simulink model "mrefrobotarm_modified_previous_y_previous_u_previous_ref_prepro"  (R2018b)
settings: Solver=FixedStepAuto  StartTime=0.0  StopTime=10  RelTol=1e-3  AbsTol=1e-6
undefined symbols (not defined in the file or in its folder): cc, options
libraries: neural x594, simulink x1
(part 18 of 22)

== system mrefrobotarm_modified_previous_y_previous_u_previous_ref_prepro/pre_0.0001/Layer 3/Delays 1 ==
  "p{3}" : Inport  PortDimensions=30
      mask Display: e = 0.06;c1 = [120 230 180]/255;c2 = ([120 230 180]+0)/(256+128);c3 = ([120 230 180]+128)/(256+128);patch([0 1 1 0],[0 0 1 1],c1);patch([0 1 1 1-e 1-e 0+e],[0 0 1 1-e 0+e 0+e],c2);patch([0 0 1 1-e 0+e 0+e],[0 1 1 1-e 1-e 0+e],c3);plot([0 1 1 0 0],[0 0 1 1 0]);
  mux : Mux  Inputs=1
      mask Display: e = 0.06;c1 = [120 150 230]/255;c2 = ([120 150 230]+0)/383;c3 = ([120 150 230]+128)/383;patch([0 1 1 0],[0 0 1 1],c1);patch([0 1 1 1-e 1-e 0+e],[0 0 1 1-e 0+e 0+e],c2);patch([0 0 1 1-e 0+e 0+e],[0 1 1 1-e 1-e 0+e],c3);plot([0 1 1 0 0],[0 0 1 1 0]);disp('Mux')
  "pd{3,2}" : Outport
      mask Display: e = 0.06;c1 = [120 230 180]/255;c2 = ([120 230 180]+0)/(256+128);c3 = ([120 230 180]+128)/(256+128);patch([0 1 1 0],[0 0 1 1],c1);patch([0 1 1 1-e 1-e 0+e],[0 0 1 1-e 0+e 0+e],c2);patch([0 0 1 1-e 0+e 0+e],[0 1 1 1-e 1-e 0+e],c3);plot([0 1 1 0 0],[0 0 1 1 0]);
  wires:
  "p{3}"/1 -> mux/1
  mux/1 -> "pd{3,2}"/1

== system mrefrobotarm_modified_previous_y_previous_u_previous_ref_prepro/pre_0.0001/Layer 3/LW{3,2} ==
  "ad{3,2}" : Inport  PortDimensions=30
      mask Display: e = 0.06;c1 = [120 230 180]/255;c2 = ([120 230 180]+0)/(256+128);c3 = ([120 230 180]+128)/(256+128);patch([0 1 1 0],[0 0 1 1],c1);patch([0 1 1 1-e 1-e 0+e],[0 0 1 1-e 0+e 0+e],c2);patch([0 0 1 1-e 0+e 0+e],[0 1 1 1-e 1-e 0+e],c3);plot([0 1 1 0 0],[0 0 1 1 0]);
  "IW{3,2}(1,:)'" : Constant  Value=[0.28550508641355853978183176877791993319988250732421875;0.1391139356255125802963590331273735500872135162353515625;-0.2200852568938792275243798712835996411740779876708984375;-0.172014640363520487920112600477295927703380584716796875;0.00622856951066873797129286316476282081566751003265380859375;-0.057862515668159801573988687550809117965400218963623046875;-0.06342329491786453943280577050245483405888080596923828125;-0.392362574699874289141376948464312590658664703369140625;-0.06328433536282289384455879144297796301543712615966796875;0.2953535370482371913425367893069051206111907958984375;-0.2194822382490898837748005689718411304056644439697265625;-0.1652625748789563198126728593706502579152584075927734375;0.17050940675530068535437067112070508301258087158203125;-0.11496607429084858276180369784924550913274288177490234375;0.19160652158000512912394697195850312709808349609375;-0.002030465333179193830603903592191272764466702938079833984375;0.05339835525288495754470119436518871225416660308837890625;-0.059270218523222110984516319831527653150260448455810546875;0.2160654531994152527385466555642778985202312469482421875;0.06461092678380074560973156394538818858563899993896484375;-0.02624333287014192495067987920265295542776584625244140625;0.04381963578903558254040717656607739627361297607421875;-0.125353371116677436702957493253052234649658203125;0.0678719790493876595771638449150486849248409271240234375;-0.1490337365498387856010964469533064402639865875244140625;0.262006071174363419640229722062940709292888641357421875;0.15556164415677808943172522049280814826488494873046875;-0.264271013352384065431266435552970506250858306884765625;0.6279513206695117588651555706746876239776611328125;-0.440731131573416534674692002226947806775569915771484375]
      mask Display: e = 0.06;c1 = [120 150 230]/255;c2 = ([120 150 230]+0)/383;c3 = ([120 150 230]+128)/383;patch([0 1 1 0],[0 0 1 1],c1);patch([0 1 1 1-e 1-e 0+e],[0 0 1 1-e 0+e 0+e],c2);patch([0 0 1 1-e 0+e 0+e],[0 1 1 1-e 1-e 0+e],c3);plot([0 1 1 0 0],[0 0 1 1 0]);disp('weights');
  Mux : Mux  Inputs=1
      mask Display: e = 0.06;c1 = [120 150 230]/255;c2 = ([120 150 230]+0)/383;c3 = ([120 150 230]+128)/383;patch([0 1 1 0],[0 0 1 1],c1);patch([0 1 1 1-e 1-e 0+e],[0 0 1 1-e 0+e 0+e],c2);patch([0 0 1 1-e 0+e 0+e],[0 1 1 1-e 1-e 0+e],c3);plot([0 1 1 0 0],[0 0 1 1 0]);disp('Mux');
  dotprod1 : neural/Weight Functions/dotprod
  "lz{3,2}" : Outport
      mask Display: e = 0.06;c1 = [120 230 180]/255;c2 = ([120 230 180]+0)/(256+128);c3 = ([120 230 180]+128)/(256+128);patch([0 1 1 0],[0 0 1 1],c1);patch([0 1 1 1-e 1-e 0+e],[0 0 1 1-e 0+e 0+e],c2);patch([0 0 1 1-e 0+e 0+e],[0 1 1 1-e 1-e 0+e],c3);plot([0 1 1 0 0],[0 0 1 1 0]);
  wires:
  "IW{3,2}(1,:)'"/1 -> dotprod1/1
  "ad{3,2}"/1 -> dotprod1/2
  dotprod1/1 -> Mux/1
  Mux/1 -> "lz{3,2}"/1

== system mrefrobotarm_modified_previous_y_previous_u_previous_ref_prepro/pre_0.001/Layer 1/Delays 1 ==
  "p{1}" : Inport  PortDimensions=10
      mask Display: e = 0.06;c1 = [120 230 180]/255;c2 = ([120 230 180]+0)/(256+128);c3 = ([120 230 180]+128)/(256+128);patch([0 1 1 0],[0 0 1 1],c1);patch([0 1 1 1-e 1-e 0+e],[0 0 1 1-e 0+e 0+e],c2);patch([0 0 1 1-e 0+e 0+e],[0 1 1 1-e 1-e 0+e],c3);plot([0 1 1 0 0],[0 0 1 1 0]);
  mux : Mux  Inputs=1
      mask Display: e = 0.06;c1 = [120 150 230]/255;c2 = ([120 150 230]+0)/383;c3 = ([120 150 230]+128)/383;patch([0 1 1 0],[0 0 1 1],c1);patch([0 1 1 1-e 1-e 0+e],[0 0 1 1-e 0+e 0+e],c2);patch([0 0 1 1-e 0+e 0+e],[0 1 1 1-e 1-e 0+e],c3);plot([0 1 1 0 0],[0 0 1 1 0]);disp('Mux')
  "pd{1,1}" : Outport
      mask Display: e = 0.06;c1 = [120 230 180]/255;c2 = ([120 230 180]+0)/(256+128);c3 = ([120 230 180]+128)/(256+128);patch([0 1 1 0],[0 0 1 1],c1);patch([0 1 1 1-e 1-e 0+e],[0 0 1 1-e 0+e 0+e],c2);patch([0 0 1 1-e 0+e 0+e],[0 1 1 1-e 1-e 0+e],c3);plot([0 1 1 0 0],[0 0 1 1 0]);
  wires:
  "p{1}"/1 -> mux/1
  mux/1 -> "pd{1,1}"/1

== system mrefrobotarm_modified_previous_y_previous_u_previous_ref_prepro/pre_0.001/Layer 1/IW{1,1} ==
  "pd{1,1}" : Inport  PortDimensions=10
      mask Display: e = 0.06;c1 = [120 230 180]/255;c2 = ([120 230 180]+0)/(256+128);c3 = ([120 230 180]+128)/(256+128);patch([0 1 1 0],[0 0 1 1],c1);patch([0 1 1 1-e 1-e 0+e],[0 0 1 1-e 0+e 0+e],c2);patch([0 0 1 1-e 0+e 0+e],[0 1 1 1-e 1-e 0+e],c3);plot([0 1 1 0 0],[0 0 1 1 0]);
  "IW{1,1}(1,:)'" : Constant  Value=[0.274177616035477356160043882482568733394145965576171875;-1.474414898369390325427730203955434262752532958984375;0.267953896034737848452778052887879312038421630859375;0.212094987555543956769810165496892295777797698974609375;-1.2502676260617338055425307175028137862682342529296875;0.5480570107188722506208478080225177109241485595703125;-0.62150052709190062305566470968187786638736724853515625;0.43047120294825436115360162148135714232921600341796875;-0.84005038898261841229242463668924756348133087158203125;0.857720533528774087272950055194087326526641845703125]
      mask Display: e = 0.06;c1 = [120 150 230]/255;c2 = ([120 150 230]+0)/383;c3 = ([120 150 230]+128)/383;patch([0 1 1 0],[0 0 1 1],c1);patch([0 1 1 1-e 1-e 0+e],[0 0 1 1-e 0+e 0+e],c2);patch([0 0 1 1-e 0+e 0+e],[0 1 1 1-e 1-e 0+e],c3);plot([0 1 1 0 0],[0 0 1 1 0]);disp('Weights');
  "IW{1,1}(10,:)'" : Constant  Value=[-0.2054329594672964220958277792306034825742244720458984375;0.5006166560364515571990295939031057059764862060546875;0.6378733309038995269446559177595190703868865966796875;-0.582428909934388006064409637474454939365386962890625;1.0631138630523242483150170301087200641632080078125;-0.9919393926062038957525146543048322200775146484375;0.3155697593642055043261507307761348783969879150390625;1.04632477637812559834173953277058899402618408203125;0.91450943731630573996227440147777087986469268798828125;0.96094358361999920870033520259312354028224945068359375]
      mask Display: e = 0.06;c1 = [120 150 230]/255;c2 = ([120 150 230]+0)/383;c3 = ([120 150 230]+128)/383;patch([0 1 1 0],[0 0 1 1],c1);patch([0 1 1 1-e 1-e 0+e],[0 0 1 1-e 0+e 0+e],c2);patch([0 0 1 1-e 0+e 0+e],[0 1 1 1-e 1-e 0+e],c3);plot([0 1 1 0 0],[0 0 1 1 0]);disp('Weights');
  "IW{1,1}(11,:)'" : Constant  Value=[0.0182200136914994932635369906392952543683350086212158203125;-0.87643721744257552241919029256678186357021331787109375;0.65626047540069887276104054762981832027435302734375;-0.9799588249276129925391387587296776473522186279296875;-0.0224161933110297896531992734026061953045427799224853515625;-1.6926058095807405834420933388173580169677734375;0.6618009923489787116324123417143709957599639892578125;-0.57104424901433337158351832840708084404468536376953125;0.451552405498240994052849828221951611340045928955078125;0.283989714346230492925116095648263581097126007080078125]
      mask Display: e = 0.06;c1 = [120 150 230]/255;c2 = ([120 150 230]+0)/383;c3 = ([120 150 230]+128)/383;patch([0 1 1 0],[0 0 1 1],c1);patch([0 1 1 1-e 1-e 0+e],[0 0 1 1-e 0+e 0+e],c2);patch([0 0 1 1-e 0+e 0+e],[0 1 1 1-e 1-e 0+e],c3);plot([0 1 1 0 0],[0 0 1 1 0]);disp('Weights');
  "IW{1,1}(12,:)'" : Constant  Value=[-0.70817734340765692291341792952152900397777557373046875;-0.491829825460522285229814087870181538164615631103515625;-0.6171636020453121762585624310304410755634307861328125;-0.93605806230037991166881283788825385272502899169921875;-1.0325649854996814536178817434119991958141326904296875;1.863897454723030033818531592260114848613739013671875;0.80757934668383857257367708371020853519439697265625;-0.15148043806354227758248498503235168755054473876953125;-1.824446524455306306577995201223529875278472900390625;-1.768122314752869073117835796438157558441162109375]
      mask Display: e = 0.06;c1 = [120 150 230]/255;c2 = ([120 150 230]+0)/383;c3 = ([120 150 230]+128)/383;patch([0 1 1 0],[0 0 1 1],c1);patch([0 1 1 1-e 1-e 0+e],[0 0 1 1-e 0+e 0+e],c2);patch([0 0 1 1-e 0+e 0+e],[0 1 1 1-e 1-e 0+e],c3);plot([0 1 1 0 0],[0 0 1 1 0]);disp('Weights');
  "IW{1,1}(13,:)'" : Constant  Value=[0.71698566688268072777390216288040392100811004638671875;1.39712735081443639728604466654360294342041015625;-0.254311878431185911519918363410397432744503021240234375;-1.4097909640270156472752205445431172847747802734375;-0.57694944863930619494141183167812414467334747314453125;1.692994982712917817480047233402729034423828125;0.2325994755679459402575304238780518062412738800048828125;0.2022436647441606394348667663507512770593166351318359375;-0.1403365846468382915901429441873915493488311767578125;-0.80876724764240270904025464915321208536624908447265625]
      mask Display: e = 0.06;c1 = [120 150 230]/255;c2 = ([120 150 230]+0)/383;c3 = ([120 150 230]+128)/383;patch([0 1 1 0],[0 0 1 1],c1);patch([0 1 1 1-e 1-e 0+e],[0 0 1 1-e 0+e 0+e],c2);patch([0 0 1 1-e 0+e 0+e],[0 1 1 1-e 1-e 0+e],c3);plot([0 1 1 0 0],[0 0 1 1 0]);disp('Weights');
  "IW{1,1}(14,:)'" : Constant  Value=[-0.635117545276415729205155003000982105731964111328125;-0.7657320958496935947579231651616282761096954345703125;-1.4346627210665394702715502717182971537113189697265625;0.67813899297114421660381822221097536385059356689453125;0.234345603011791692171783552112174220383167266845703125;0.66374486654939601759650713574956171214580535888671875;-0.62994783335228887732881730698863975703716278076171875;0.48210259229915297662927287092315964400768280029296875;0.4351347373171734478347616459359414875507354736328125;-1.298038422264415903129020080086775124073028564453125]
      mask Display: e = 0.06;c1 = [120 150 230]/255;c2 = ([120 150 230]+0)/383;c3 = ([120 150 230]+128)/383;patch([0 1 1 0],[0 0 1 1],c1);patch([0 1 1 1-e 1-e 0+e],[0 0 1 1-e 0+e 0+e],c2);patch([0 0 1 1-e 0+e 0+e],[0 1 1 1-e 1-e 0+e],c3);plot([0 1 1 0 0],[0 0 1 1 0]);disp('Weights');
  "IW{1,1}(15,:)'" : Constant  Value=[0.615520126635521247493443297571502625942230224609375;-0.296207622798284386789191557909362018108367919921875;0.440297608285253605497899798137950710952281951904296875;-0.29755007333499483568317600656882859766483306884765625;0.9039031279234903681896184934885241091251373291015625;-1.8383313614436342930957835051231086254119873046875;-0.2223865940820675124456329285749234259128570556640625;0.84459071589224266052298162321676500141620635986328125;1.20007646223651409655985844437964260578155517578125;1.956422886115234405224327929317951202392578125]
      mask Display: e = 0.06;c1 = [120 150 230]/255;c2 = ([120 150 230]+0)/383;c3 = ([120 150 230]+128)/383;patch([0 1 1 0],[0 0 1 1],c1);patch([0 1 1 1-e 1-e 0+e],[0 0 1 1-e 0+e 0+e],c2);patch([0 0 1 1-e 0+e 0+e],[0 1 1 1-e 1-e 0+e],c3);plot([0 1 1 0 0],[0 0 1 1 0]);disp('Weights');
  "IW{1,1}(16,:)'" : Constant  Value=[0.6777102116673159315496377530507743358612060546875;-0.1055782839275415663227164486670517362654209136962890625;0.74321951112662387739504765704623423516750335693359375;-0.477203795335321145909546203256468288600444793701171875;1.411313293363029242044603961403481662273406982421875;-1.3888516734461517909693384353886358439922332763671875;1.461924656924883603181797298020683228969573974609375;-0.50256057571066736766596250163274817168712615966796875;1.76242589468333932245514006353914737701416015625;-0.444898203177669870900245996381272561848163604736328125]
      mask Display: e = 0.06;c1 = [120 150 230]/255;c2 = ([120 150 230]+0)/383;c3 = ([120 150 230]+128)/383;patch([0 1 1 0],[0 0 1 1],c1);patch([0 1 1 1-e 1-e 0+e],[0 0 1 1-e 0+e 0+e],c2);patch([0 0 1 1-e 0+e 0+e],[0 1 1 1-e 1-e 0+e],c3);plot([0 1 1 0 0],[0 0 1 1 0]);disp('Weights');
  "IW{1,1}(17,:)'" : Constant  Value=[0.59831518582436860054230010064202360808849334716796875;0.87213059943941007023937572739669121801853179931640625;-0.481679760061163697582031772981281392276287078857421875;0.27724517901343437298322669448680244386196136474609375;-0.31799033477524429880389789104810915887355804443359375;1.4309306759273663356424322046223096549510955810546875;-0.501280177699635398624877780093811452388763427734375;0.5183389231116135587029702946892939507961273193359375;1.01138633319924498010777824674732983112335205078125;-0.9155537494118457519931553179048933088779449462890625]
      mask Display: e = 0.06;c1 = [120 150 230]/255;c2 = ([120 150 230]+0)/383;c3 = ([120 150 230]+128)/383;patch([0 1 1 0],[0 0 1 1],c1);patch([0 1 1 1-e 1-e 0+e],[0 0 1 1-e 0+e 0+e],c2);patch([0 0 1 1-e 0+e 0+e],[0 1 1 1-e 1-e 0+e],c3);plot([0 1 1 0 0],[0 0 1 1 0]);disp('Weights');
  "IW{1,1}(18,:)'" : Constant  Value=[0.496452254621586153149337405920960009098052978515625;-0.456951622552531910859130448443465866148471832275390625;-0.2068080558972722748922734581356053240597248077392578125;-0.66171061135404285469263641061843372881412506103515625;0.92387478830275016061790438470779918134212493896484375;0.90185966971914499623608207912184298038482666015625;0.84472318010530000886859625097713433206081390380859375;-0.96889912783830778320037779849371872842311859130859375;1.1840076074866521249617790090269409120082855224609375;1.6327096000134790898528081015683710575103759765625]
      mask Display: e = 0.06;c1 = [120 150 230]/255;c2 = ([120 150 230]+0)/383;c3 = ([120 150 230]+128)/383;patch([0 1 1 0],[0 0 1 1],c1);patch([0 1 1 1-e 1-e 0+e],[0 0 1 1-e 0+e 0+e],c2);patch([0 0 1 1-e 0+e 0+e],[0 1 1 1-e 1-e 0+e],c3);plot([0 1 1 0 0],[0 0 1 1 0]);disp('Weights');
  "IW{1,1}(19,:)'" : Constant  Value=[0.59854544548408872284284143461263738572597503662109375;0.97946811048223947349100626524887047708034515380859375;0.09928491978776683712926143243748811073601245880126953125;-1.9556761744024704352540311447228305041790008544921875;-0.45457767176392704921994436517707072198390960693359375;-0.3051524474728946056956147003802470862865447998046875;1.4305577520598280472086116787977516651153564453125;1.2585088615100412656744310879730619490146636962890625;-0.012590455091918521801641617230416159145534038543701171875;-1.0849803780911475570292168413288891315460205078125]
      mask Display: e = 0.06;c1 = [120 150 230]/255;c2 = ([120 150 230]+0)/383;c3 = ([120 150 230]+128)/383;patch([0 1 1 0],[0 0 1 1],c1);patch([0 1 1 1-e 1-e 0+e],[0 0 1 1-e 0+e 0+e],c2);patch([0 0 1 1-e 0+e 0+e],[0 1 1 1-e 1-e 0+e],c3);plot([0 1 1 0 0],[0 0 1 1 0]);disp('Weights');
  "IW{1,1}(2,:)'" : Constant  Value=[0.0504117522830804798417148049338720738887786865234375;0.46063276814139386683422117130248807370662689208984375;0.487357149222266750054899375754757784307003021240234375;-0.32788144850375833261324487466481514275074005126953125;-0.68029452669381351714861239088349975645542144775390625;-1.018017187298617454160876150126568973064422607421875;0.01184893335260418789633973801755928434431552886962890625;0.80520378022615857194210775560350157320499420166015625;-1.250982961123832115646337115322239696979522705078125;-0.1428040247193382017432128350264974869787693023681640625]
      mask Display: e = 0.06;c1 = [120 150 230]/255;c2 = ([120 150 230]+0)/383;c3 = ([120 150 230]+128)/383;patch([0 1 1 0],[0 0 1 1],c1);patch([0 1 1 1-e 1-e 0+e],[0 0 1 1-e 0+e 0+e],c2);patch([0 0 1 1-e 0+e 0+e],[0 1 1 1-e 1-e 0+e],c3);plot([0 1 1 0 0],[0 0 1 1 0]);disp('Weights');
  "IW{1,1}(20,:)'" : Constant  Value=[-0.44391799480924010179450078794616274535655975341796875;0.569327047589569534835618469514884054660797119140625;-1.094181999161283780352960093296132981777191162109375;0.62416680247855216290275848223245702683925628662109375;1.189632572385828979122379678301513195037841796875;-2.2646036580378989810924394987523555755615234375;0.469618036158499674304067639241111464798450469970703125;0.348029724788706806837268459275946952402591705322265625;-1.1797505009561233269010926960618235170841217041015625;1.004054492112516516755249540437944233417510986328125]
      mask Display: e = 0.06;c1 = [120 150 230]/255;c2 = ([120 150 230]+0)/383;c3 = ([120 150 230]+128)/383;patch([0 1 1 0],[0 0 1 1],c1);patch([0 1 1 1-e 1-e 0+e],[0 0 1 1-e 0+e 0+e],c2);patch([0 0 1 1-e 0+e 0+e],[0 1 1 1-e 1-e 0+e],c3);plot([0 1 1 0 0],[0 0 1 1 0]);disp('Weights');
  "IW{1,1}(21,:)'" : Constant  Value=[-0.06307210773920253477076158787895110435783863067626953125;-0.493331013996436140711665530034224502742290496826171875;-0.007596442328687978869095065448391324025578796863555908203125;1.1099941867034293085936269562807865440845489501953125;-2.045172848482042393669644297915510833263397216796875;1.3071313538333415582570751212188042700290679931640625;-0.07772567333255812893622049841724219731986522674560546875;-1.534434562569752191762972870492376387119293212890625;0.483545075650703759517767821307643316686153411865234375;0.369808475546980319759171607074677012860774993896484375]
      mask Display: e = 0.06;c1 = [120 150 230]/255;c2 = ([120 150 230]+0)/383;c3 = ([120 150 230]+128)/383;patch([0 1 1 0],[0 0 1 1],c1);patch([0 1 1 1-e 1-e 0+e],[0 0 1 1-e 0+e 0+e],c2);patch([0 0 1 1-e 0+e 0+e],[0 1 1 1-e 1-e 0+e],c3);plot([0 1 1 0 0],[0 0 1 1 0]);disp('Weights');
  "IW{1,1}(22,:)'" : Constant  Value=[0.466818152502863459307747007187572307884693145751953125;-0.73811697103160234245677884246106259524822235107421875;0.027333155768829386911278334082453511655330657958984375;0.284365738169115978006828981961007229983806610107421875;0.235945222693785650047715307664475403726100921630859375;0.12358213210766884337932225434997235424816608428955078125;1.41248443007588786457517926464788615703582763671875;-0.1257822294110042538051175142754800617694854736328125;1.56979626746996103747733286581933498382568359375;0.1968076429879257183142016174315358512103557586669921875]
      mask Display: e = 0.06;c1 = [120 150 230]/255;c2 = ([120 150 230]+0)/383;c3 = ([120 150 230]+128)/383;patch([0 1 1 0],[0 0 1 1],c1);patch([0 1 1 1-e 1-e 0+e],[0 0 1 1-e 0+e 0+e],c2);patch([0 0 1 1-e 0+e 0+e],[0 1 1 1-e 1-e 0+e],c3);plot([0 1 1 0 0],[0 0 1 1 0]);disp('Weights');
  "IW{1,1}(23,:)'" : Constant  Value=[0.234666638593052756522894242152688093483448028564453125;0.485568510336121084147720239343470893800258636474609375;0.73005002203585667164276173934922553598880767822265625;-0.266174706769144953089067939799861051142215728759765625;-1.8925808014698544123888268586597405374050140380859375;1.103451881369226672546801637508906424045562744140625;0.2574468976701413946983620917308144271373748779296875;-0.21158458097743781944899410518701188266277313232421875;0.1200039715087337921506360771672916598618030548095703125;-0.1996850401149956322210954340334865264594554901123046875]
      mask Display: e = 0.06;c1 = [120 150 230]/255;c2 = ([120 150 230]+0)/383;c3 = ([120 150 230]+128)/383;patch([0 1 1 0],[0 0 1 1],c1);patch([0 1 1 1-e 1-e 0+e],[0 0 1 1-e 0+e 0+e],c2);patch([0 0 1 1-e 0+e 0+e],[0 1 1 1-e 1-e 0+e],c3);plot([0 1 1 0 0],[0 0 1 1 0]);disp('Weights');
  "IW{1,1}(24,:)'" : Constant  Value=[-0.7551447567828744045215216829092241823673248291015625;0.360507980565289931629280317793018184602260589599609375;-0.5368451752868022008868820194038562476634979248046875;0.9419086159752716458370969121460802853107452392578125;1.4589739906700989191534745259559713304042816162109375;-1.6780485996799898718023769106366671621799468994140625;-0.447862965351764064081407923367805778980255126953125;-0.81510579016904916027641547771054320037364959716796875;0.444657465454466827026180908433161675930023193359375;0.3315952933723955720068943264777772128582000732421875]
      mask Display: e = 0.06;c1 = [120 150 230]/255;c2 = ([120 150 230]+0)/383;c3 = ([120 150 230]+128)/383;patch([0 1 1 0],[0 0 1 1],c1);patch([0 1 1 1-e 1-e 0+e],[0 0 1 1-e 0+e 0+e],c2);patch([0 0 1 1-e 0+e 0+e],[0 1 1 1-e 1-e 0+e],c3);plot([0 1 1 0 0],[0 0 1 1 0]);disp('Weights');
  "IW{1,1}(25,:)'" : Constant  Value=[0.52191338596319436504700206569395959377288818359375;-0.2931240241627770526378071735962294042110443115234375;-0.271642625897154876835060122175491414964199066162109375;0.78846776965071063703049958348856307566165924072265625;0.396604381772453551402435323325335048139095306396484375;-1.315302459142093649546723099774681031703948974609375;0.5316363118649400920645575752132572233676910400390625;0.148558274035188342399038674557232297956943511962890625;-1.7136871556689998730149682160117663443088531494140625;-1.170883904641701889204341568984091281890869140625]
      mask Display: e = 0.06;c1 = [120 150 230]/255;c2 = ([120 150 230]+0)/383;c3 = ([120 150 230]+128)/383;patch([0 1 1 0],[0 0 1 1],c1);patch([0 1 1 1-e 1-e 0+e],[0 0 1 1-e 0+e 0+e],c2);patch([0 0 1 1-e 0+e 0+e],[0 1 1 1-e 1-e 0+e],c3);plot([0 1 1 0 0],[0 0 1 1 0]);disp('Weights');
  "IW{1,1}(26,:)'" : Constant  Value=[0.50274305848446509958904471204732544720172882080078125;0.36148475686855874311476100047002546489238739013671875;0.411401540080265692989058834427851252257823944091796875;0.29112781501617368551393383313552476465702056884765625;1.912714135105971546835235130856744945049285888671875;-1.25837903103114445713117675040848553180694580078125;-1.0869614322661476091269605603883974254131317138671875;0.6051088148574395031431549796252511441707611083984375;0.25753603468957642075309877327526919543743133544921875;-0.52829238933861122351487438209005631506443023681640625]
      mask Display: e = 0.06;c1 = [120 150 230]/255;c2 = ([120 150 230]+0)/383;c3 = ([120 150 230]+128)/383;patch([0 1 1 0],[0 0 1 1],c1);patch([0 1 1 1-e 1-e 0+e],[0 0 1 1-e 0+e 0+e],c2);patch([0 0 1 1-e 0+e 0+e],[0 1 1 1-e 1-e 0+e],c3);plot([0 1 1 0 0],[0 0 1 1 0]);disp('Weights');
  "IW{1,1}(27,:)'" : Constant  Value=[0.20909910907242068578426597014185972511768341064453125;-1.1201810396949973824831658930634148418903350830078125;-0.61169217100969586198289107414893805980682373046875;0.63324534665924658849434081275830976665019989013671875;1.12279324323989637690601739450357854366302490234375;1.2618057946744081210255217229132540524005889892578125;-0.46321642205946178538766844212659634649753570556640625;0.002391197888603675304752815833353452035225927829742431640625;-0.205421992642841277909582231586682610213756561279296875;0.486463094990449373966612256481312215328216552734375]
      mask Display: e = 0.06;c1 = [120 150 230]/255;c2 = ([120 150 230]+0)/383;c3 = ([120 150 230]+128)/383;patch([0 1 1 0],[0 0 1 1],c1);patch([0 1 1 1-e 1-e 0+e],[0 0 1 1-e 0+e 0+e],c2);patch([0 0 1 1-e 0+e 0+e],[0 1 1 1-e 1-e 0+e],c3);plot([0 1 1 0 0],[0 0 1 1 0]);disp('Weights');
  "IW{1,1}(28,:)'" : Constant  Value=[0.5434680001554870187874257680959999561309814453125;0.077352570614491467093642995678237639367580413818359375;0.390839152793104827043890736604225821793079376220703125;-0.2359203153763977656165451435299473814666271209716796875;0.8681939165048662143675528568564914166927337646484375;-0.28279697895913080696317365436698310077190399169921875;0.2616586706808756712661079291137866675853729248046875;0.801928316315346112475026529864408075809478759765625;0.946114901619230064255816614604555070400238037109375;0.79850575792669242769505899559590034186840057373046875]
      mask Display: e = 0.06;c1 = [120 150 230]/255;c2 = ([120 150 230]+0)/383;c3 = ([120 150 230]+128)/383;patch([0 1 1 0],[0 0 1 1],c1);patch([0 1 1 1-e 1-e 0+e],[0 0 1 1-e 0+e 0+e],c2);patch([0 0 1 1-e 0+e 0+e],[0 1 1 1-e 1-e 0+e],c3);plot([0 1 1 0 0],[0 0 1 1 0]);disp('Weights');
  "IW{1,1}(29,:)'" : Constant  Value=[0.266283067344181223479182563096401281654834747314453125;0.81963033079652014567528794941608794033527374267578125;0.06733545885411278131282841741267475299537181854248046875;-0.5376438044739939581262433421215973794460296630859375;1.4013291918193300222839070556801743805408477783203125;-0.2995982498436531304975005696178413927555084228515625;-0.58188123793987733822774544023559428751468658447265625;0.5189855381620007701570784774958156049251556396484375;0.5828681714830958870976473917835392057895660400390625;-1.35856450375826920407007492030970752239227294921875]
      mask Display: e = 0.06;c1 = [120 150 230]/255;c2 = ([120 150 230]+0)/383;c3 = ([120 150 230]+128)/383;patch([0 1 1 0],[0 0 1 1],c1);patch([0 1 1 1-e 1-e 0+e],[0 0 1 1-e 0+e 0+e],c2);patch([0 0 1 1-e 0+e 0+e],[0 1 1 1-e 1-e 0+e],c3);plot([0 1 1 0 0],[0 0 1 1 0]);disp('Weights');
  "IW{1,1}(3,:)'" : Constant  Value=[-0.04125436580616635706686423645805916748940944671630859375;-1.1497842171766252672426844583242200314998626708984375;0.3200714406333349248967579114832915365695953369140625;0.0695085308815579228092218500023591332137584686279296875;1.0981655363692859328494932924513705074787139892578125;-0.53742025618871147596422588321729563176631927490234375;1.803341603701569706430518635897897183895111083984375;0.453951491140188789774612132532638497650623321533203125;1.573794384082385366951939431601203978061676025390625;-0.15201564513826593127987507614307105541229248046875]
      mask Display: e = 0.06;c1 = [120 150 230]/255;c2 = ([120 150 230]+0)/383;c3 = ([120 150 230]+128)/383;patch([0 1 1 0],[0 0 1 1],c1);patch([0 1 1 1-e 1-e 0+e],[0 0 1 1-e 0+e 0+e],c2);patch([0 0 1 1-e 0+e 0+e],[0 1 1 1-e 1-e 0+e],c3);plot([0 1 1 0 0],[0 0 1 1 0]);disp('Weights');
  "IW{1,1}(30,:)'" : Constant  Value=[-0.12168897402325896950348038672018446959555149078369140625;-1.4628404096465079664568520456668920814990997314453125;0.1004828823907444601548633045240421779453754425048828125;-0.79664951511072790157896861273911781609058380126953125;3.10940162718103696448679329478181898593902587890625;-2.073267011275338855824657002813182771205902099609375;0.36014735729113100948239889476099051535129547119140625;0.12297719537435958248039469253853894770145416259765625;0.75688473681449985885905107352300547063350677490234375;-0.43248746722462783065310532037983648478984832763671875]
      mask Display: e = 0.06;c1 = [120 150 230]/255;c2 = ([120 150 230]+0)/383;c3 = ([120 150 230]+128)/383;patch([0 1 1 0],[0 0 1 1],c1);patch([0 1 1 1-e 1-e 0+e],[0 0 1 1-e 0+e 0+e],c2);patch([0 0 1 1-e 0+e 0+e],[0 1 1 1-e 1-e 0+e],c3);plot([0 1 1 0 0],[0 0 1 1 0]);disp('Weights');
  "IW{1,1}(4,:)'" : Constant  Value=[-0.5777513068741957358298577673849649727344512939453125;0.991917608781715642862764070741832256317138671875;-0.494269989190201430862003917354741133749485015869140625;-0.78532754156830841818504040929838083684444427490234375;-1.1633542371681635518854136535082943737506866455078125;-0.92587414036949200468740173164405860006809234619140625;-0.19795261026205490662022157266619615256786346435546875;0.85666639425335378010828435435541905462741851806640625;-0.433060155105392141638986913676490075886249542236328125;0.1961773577788645528396926920322584919631481170654296875]
      mask Display: e = 0.06;c1 = [120 150 230]/255;c2 = ([120 150 230]+0)/383;c3 = ([120 150 230]+128)/383;patch([0 1 1 0],[0 0 1 1],c1);patch([0 1 1 1-e 1-e 0+e],[0 0 1 1-e 0+e 0+e],c2);patch([0 0 1 1-e 0+e 0+e],[0 1 1 1-e 1-e 0+e],c3);plot([0 1 1 0 0],[0 0 1 1 0]);disp('Weights');
  "IW{1,1}(5,:)'" : Constant  Value=[0.09795788229359592147460489286459051072597503662109375;-0.77874382382369644606256997576565481722354888916015625;-0.10095311030559687981433825143540161661803722381591796875;-0.02666970541520748139152630074022454209625720977783203125;1.7693134621034880549217405132367275655269622802734375;-0.615071478078454969562471887911669909954071044921875;-0.9439983441786592432976021882495842874050140380859375;-1.2813072122858901735753534012474119663238525390625;-1.0672554353891172684853927421499975025653839111328125;-0.45212759354588072380209951006690971553325653076171875]
      mask Display: e = 0.06;c1 = [120 150 230]/255;c2 = ([120 150 230]+0)/383;c3 = ([120 150 230]+128)/383;patch([0 1 1 0],[0 0 1 1],c1);patch([0 1 1 1-e 1-e 0+e],[0 0 1 1-e 0+e 0+e],c2);patch([0 0 1 1-e 0+e 0+e],[0 1 1 1-e 1-e 0+e],c3);plot([0 1 1 0 0],[0 0 1 1 0]);disp('Weights');
  "IW{1,1}(6,:)'" : Constant  Value=[0.284943138137430496126256684874533675611019134521484375;-0.85716100877836820526312067158869467675685882568359375;-1.3688674915611744875576505364733748137950897216796875;-0.459702214220590377191655306887696497142314910888671875;0.4513939952402894473237893180339597165584564208984375;0.1461403762495152858225111458523315377533435821533203125;-0.9017862573439874296354901161976158618927001953125;0.431155987860699474456538382582948543131351470947265625;-0.1784314305859067972814813174409209750592708587646484375;0.3633235183791565514610510945203714072704315185546875]
      mask Display: e = 0.06;c1 = [120 150 230]/255;c2 = ([120 150 230]+0)/383;c3 = ([120 150 230]+128)/383;patch([0 1 1 0],[0 0 1 1],c1);patch([0 1 1 1-e 1-e 0+e],[0 0 1 1-e 0+e 0+e],c2);patch([0 0 1 1-e 0+e 0+e],[0 1 1 1-e 1-e 0+e],c3);plot([0 1 1 0 0],[0 0 1 1 0]);disp('Weights');
  "IW{1,1}(7,:)'" : Constant  Value=[0.81599575134368362849812683634809218347072601318359375;0.455748225762320213760858678142540156841278076171875;1.0855237938633106598018684962880797684192657470703125;-0.825532746992510002570497817941941320896148681640625;1.0432753490999269185834918971522711217403411865234375;1.1150123722211724430763979398761875927448272705078125;-2.307124673511701029582354749436490237712860107421875;-0.2096799086152394131499221430203760974109172821044921875;-0.4690524779182023706880499958060681819915771484375;0.8914423768784747181825878215022385120391845703125]
      mask Display: e = 0.06;c1 = [120 150 230]/255;c2 = ([120 150 230]+0)/383;c3 = ([120 150 230]+128)/383;patch([0 1 1 0],[0 0 1 1],c1);patch([0 1 1 1-e 1-e 0+e],[0 0 1 1-e 0+e 0+e],c2);patch([0 0 1 1-e 0+e 0+e],[0 1 1 1-e 1-e 0+e],c3);plot([0 1 1 0 0],[0 0 1 1 0]);disp('Weights');
  "IW{1,1}(8,:)'" : Constant  Value=[-0.3625704449393849504446052378625608980655670166015625;0.9143392237245306919390941402525641024112701416015625;-0.1918229145086700893063635930957389064133167266845703125;-0.417128149483867283198179620740120299160480499267578125;1.757561379448855820584185494226403534412384033203125;-0.82644571435967051353799206481198780238628387451171875;-1.16777874231987510711405775509774684906005859375;0.6859748182186056197906509623862802982330322265625;0.257329657955757351572856350685469806194305419921875;-1.340617856720728529040798093774355947971343994140625]
      mask Display: e = 0.06;c1 = [120 150 230]/255;c2 = ([120 150 230]+0)/383;c3 = ([120 150 230]+128)/383;patch([0 1 1 0],[0 0 1 1],c1);patch([0 1 1 1-e 1-e 0+e],[0 0 1 1-e 0+e 0+e],c2);patch([0 0 1 1-e 0+e 0+e],[0 1 1 1-e 1-e 0+e],c3);plot([0 1 1 0 0],[0 0 1 1 0]);disp('Weights');
  "IW{1,1}(9,:)'" : Constant  Value=[0.8725528454636604092087281969725154340267181396484375;0.0154371974622351804118380869113025255501270294189453125;0.2458687717231116398597379202328738756477832794189453125;-0.79184799756538259973837057259515859186649322509765625;0.752302594824351356095348819508217275142669677734375;-2.61048516472820946177080259076319634914398193359375;-1.3322787332551666583668747989577241241931915283203125;1.2965377006275262683487881076871417462825775146484375;0.57696631009189214278620738696190528571605682373046875;-0.51149227507034955575448975650942884385585784912109375]
      mask Display: e = 0.06;c1 = [120 150 230]/255;c2 = ([120 150 230]+0)/383;c3 = ([120 150 230]+128)/383;patch([0 1 1 0],[0 0 1 1],c1);patch([0 1 1 1-e 1-e 0+e],[0 0 1 1-e 0+e 0+e],c2);patch([0 0 1 1-e 0+e 0+e],[0 1 1 1-e 1-e 0+e],c3);plot([0 1 1 0 0],[0 0 1 1 0]);disp('Weights');
  Mux : Mux  Inputs=30
      mask Display: e = 0.06;c1 = [120 150 230]/255;c2 = ([120 150 230]+0)/383;c3 = ([120 150 230]+128)/383;patch([0 1 1 0],[0 0 1 1],c1);patch([0 1 1 1-e 1-e 0+e],[0 0 1 1-e 0+e 0+e],c2);patch([0 0 1 1-e 0+e 0+e],[0 1 1 1-e 1-e 0+e],c3);plot([0 1 1 0 0],[0 0 1 1 0]);disp('Mux');
  dotprod{1..30} (30 alike) : neural/Weight Functions/dotprod
  "iz{1,1}" : Outport
      mask Display: e = 0.06;c1 = [120 230 180]/255;c2 = ([120 230 180]+0)/(256+128);c3 = ([120 230 180]+128)/(256+128);patch([0 1 1 0],[0 0 1 1],c1);patch([0 1 1 1-e 1-e 0+e],[0 0 1 1-e 0+e 0+e],c2);patch([0 0 1 1-e 0+e 0+e],[0 1 1 1-e 1-e 0+e],c3);plot([0 1 1 0 0],[0 0 1 1 0]);
  wires:
  "IW{1,1}(1,:)'"/1 -> dotprod1/1
  "pd{1,1}"/1 -> dotprod1/2, dotprod2/2, dotprod3/2, dotprod4/2, dotprod5/2, dotprod6/2, dotprod7/2, dotprod8/2, dotprod9/2, dotprod10/2, dotprod11/2, dotprod12/2, dotprod13/2, dotprod14/2, dotprod15/2, dotprod16/2, dotprod17/2, dotprod18/2, dotprod19/2, dotprod20/2, dotprod21/2, dotprod22/2, dotprod23/2, dotprod24/2, dotprod25/2, dotprod26/2, dotprod27/2, dotprod28/2, dotprod29/2, dotprod30/2
  dotprod1/1 -> Mux/1
  "IW{1,1}(2,:)'"/1 -> dotprod2/1
  dotprod2/1 -> Mux/2
  "IW{1,1}(3,:)'"/1 -> dotprod3/1
  dotprod3/1 -> Mux/3
  "IW{1,1}(4,:)'"/1 -> dotprod4/1
  dotprod4/1 -> Mux/4
  "IW{1,1}(5,:)'"/1 -> dotprod5/1
  dotprod5/1 -> Mux/5
  "IW{1,1}(6,:)'"/1 -> dotprod6/1
  dotprod6/1 -> Mux/6
  "IW{1,1}(7,:)'"/1 -> dotprod7/1
  dotprod7/1 -> Mux/7
  "IW{1,1}(8,:)'"/1 -> dotprod8/1
  dotprod8/1 -> Mux/8
  "IW{1,1}(9,:)'"/1 -> dotprod9/1
  dotprod9/1 -> Mux/9
  "IW{1,1}(10,:)'"/1 -> dotprod10/1
  dotprod10/1 -> Mux/10
  "IW{1,1}(11,:)'"/1 -> dotprod11/1
  dotprod11/1 -> Mux/11
  "IW{1,1}(12,:)'"/1 -> dotprod12/1
  dotprod12/1 -> Mux/12
  "IW{1,1}(13,:)'"/1 -> dotprod13/1
  dotprod13/1 -> Mux/13
  "IW{1,1}(14,:)'"/1 -> dotprod14/1
  dotprod14/1 -> Mux/14
  "IW{1,1}(15,:)'"/1 -> dotprod15/1
  dotprod15/1 -> Mux/15
  "IW{1,1}(16,:)'"/1 -> dotprod16/1
  dotprod16/1 -> Mux/16
  "IW{1,1}(17,:)'"/1 -> dotprod17/1
  dotprod17/1 -> Mux/17
  "IW{1,1}(18,:)'"/1 -> dotprod18/1
  dotprod18/1 -> Mux/18
  "IW{1,1}(19,:)'"/1 -> dotprod19/1
  dotprod19/1 -> Mux/19
  "IW{1,1}(20,:)'"/1 -> dotprod20/1
  dotprod20/1 -> Mux/20
  "IW{1,1}(21,:)'"/1 -> dotprod21/1
  dotprod21/1 -> Mux/21
  "IW{1,1}(22,:)'"/1 -> dotprod22/1
  dotprod22/1 -> Mux/22
  "IW{1,1}(23,:)'"/1 -> dotprod23/1
  dotprod23/1 -> Mux/23
  "IW{1,1}(24,:)'"/1 -> dotprod24/1
  dotprod24/1 -> Mux/24
  "IW{1,1}(25,:)'"/1 -> dotprod25/1
  dotprod25/1 -> Mux/25
  "IW{1,1}(26,:)'"/1 -> dotprod26/1
  dotprod26/1 -> Mux/26
  "IW{1,1}(27,:)'"/1 -> dotprod27/1
  dotprod27/1 -> Mux/27
  "IW{1,1}(28,:)'"/1 -> dotprod28/1
  dotprod28/1 -> Mux/28
  "IW{1,1}(29,:)'"/1 -> dotprod29/1
  dotprod29/1 -> Mux/29
  "IW{1,1}(30,:)'"/1 -> dotprod30/1
  dotprod30/1 -> Mux/30
  Mux/1 -> "iz{1,1}"/1

== system mrefrobotarm_modified_previous_y_previous_u_previous_ref_prepro/pre_0.001/Layer 2/Delays 1 ==
  "p{2}" : Inport  PortDimensions=30
      mask Display: e = 0.06;c1 = [120 230 180]/255;c2 = ([120 230 180]+0)/(256+128);c3 = ([120 230 180]+128)/(256+128);patch([0 1 1 0],[0 0 1 1],c1);patch([0 1 1 1-e 1-e 0+e],[0 0 1 1-e 0+e 0+e],c2);patch([0 0 1 1-e 0+e 0+e],[0 1 1 1-e 1-e 0+e],c3);plot([0 1 1 0 0],[0 0 1 1 0]);
  mux : Mux  Inputs=1
      mask Display: e = 0.06;c1 = [120 150 230]/255;c2 = ([120 150 230]+0)/383;c3 = ([120 150 230]+128)/383;patch([0 1 1 0],[0 0 1 1],c1);patch([0 1 1 1-e 1-e 0+e],[0 0 1 1-e 0+e 0+e],c2);patch([0 0 1 1-e 0+e 0+e],[0 1 1 1-e 1-e 0+e],c3);plot([0 1 1 0 0],[0 0 1 1 0]);disp('Mux')
  "pd{2,1}" : Outport
      mask Display: e = 0.06;c1 = [120 230 180]/255;c2 = ([120 230 180]+0)/(256+128);c3 = ([120 230 180]+128)/(256+128);patch([0 1 1 0],[0 0 1 1],c1);patch([0 1 1 1-e 1-e 0+e],[0 0 1 1-e 0+e 0+e],c2);patch([0 0 1 1-e 0+e 0+e],[0 1 1 1-e 1-e 0+e],c3);plot([0 1 1 0 0],[0 0 1 1 0]);
  wires:
  "p{2}"/1 -> mux/1
  mux/1 -> "pd{2,1}"/1
